simulink model "UAV_simple_hw_architecture"  (R2021b)
settings: Solver=VariableStepAuto  StartTime=0.0  StopTime=10.0  RelTol=1e-3
model workspace (MAT data in the model file):
  sensorData = Simulink.Bus
  sensorData.Alignment = -1
  sensorData.PreserveElementDimensions = 0
  sensorData.DataScope = 'Auto'
settings Model: Creator=esther  LastModifiedBy=esther

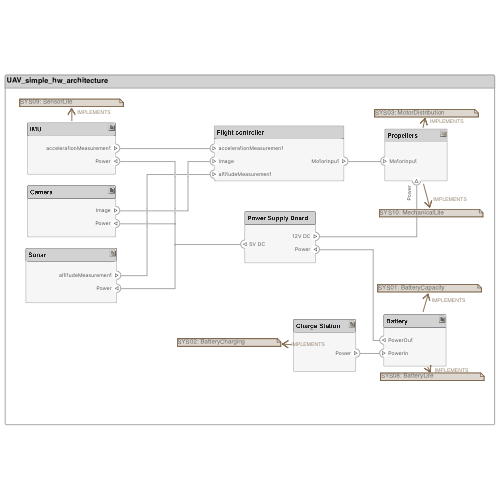
[thumbnail: Simulink's stored preview of the top-level diagram]
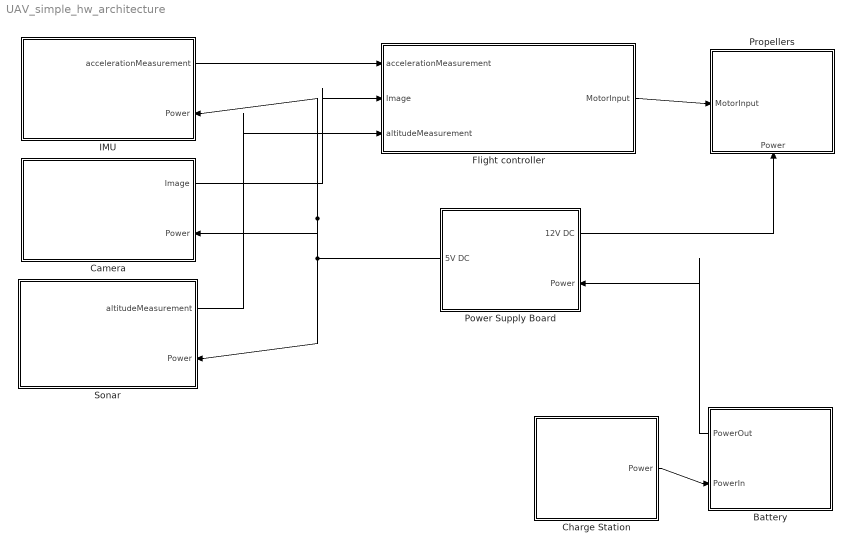
== system UAV_simple_hw_architecture ==
  Battery : Subsystem
      settings: PortSchema="{\"entries\":[{\"content\":{\"headerSize\":26,\"margin\":15,\"minimumSpacing\":25,\"sides\":[{\"content\":{\"connectorIds\":[\"Out1\",\"In1\"]},\"type\":\"ConnectorPlacement.EquallySpacedRectSide\",\"uuid\":\"982650e6-ddcc-430e-b118-190f1a8c1bc9\"},{\"content\":{\"connectorIds\":[],\"side\":\"RIGHT\"},\"type\":\"ConnectorPlacement.EquallySpacedRectSide\",\"uuid\":\"ed844e2c-e9bb-41b6-92bb-7e682fbb84b4\"},{\"content\":{\"connectorIds\":[],\"side\":\"TOP\"},\"type\":\"ConnectorPlacement.EquallySpacedRectSide\",\"uuid\":\"fdc513b0-7393-49dc-b7da-10bb51e0d5fd\"},{\"content\":{\"connectorIds\":[],\"side\":\"BOTTOM\"},\"type\":\"ConnectorPlacement.EquallySpacedRectSide\",\"uuid\":\"d8953aff-5649-44c5-a700-2c484cd66d11\"}]},\"type\":\"ConnectorPlacement.EquallySpacedConnector\",\"uuid\":\"3b6a0f0d-75bf-4e75-a7db-e0984288cb82\"}],\"packageUris\":[\"http://schema.mathworks.com/mf0/Connector/R2020b\"],\"version\":\"1.0\"}"
  Camera : Subsystem
      settings: PortSchema="{\"entries\":[{\"content\":{\"headerSize\":26,\"margin\":15,\"minimumSpacing\":25,\"sides\":[{\"content\":{\"connectorIds\":[]},\"type\":\"ConnectorPlacement.EquallySpacedRectSide\",\"uuid\":\"982650e6-ddcc-430e-b118-190f1a8c1bc9\"},{\"content\":{\"connectorIds\":[\"Out1\",\"In1\"],\"side\":\"RIGHT\"},\"type\":\"ConnectorPlacement.EquallySpacedRectSide\",\"uuid\":\"ed844e2c-e9bb-41b6-92bb-7e682fbb84b4\"},{\"content\":{\"connectorIds\":[],\"side\":\"TOP\"},\"type\":\"ConnectorPlacement.EquallySpacedRectSide\",\"uuid\":\"fdc513b0-7393-49dc-b7da-10bb51e0d5fd\"}]},\"type\":\"ConnectorPlacement.EquallySpacedConnector\",\"uuid\":\"3b6a0f0d-75bf-4e75-a7db-e0984288cb82\"}],\"packageUris\":[\"http://schema.mathworks.com/mf0/Connector/R2020b\"],\"version\":\"1.0\"}"
  Charge Station : Subsystem
      settings: PortSchema="{\"entries\":[{\"content\":{\"headerSize\":26,\"margin\":15,\"minimumSpacing\":25,\"sides\":[{\"content\":{\"connectorIds\":[]},\"type\":\"ConnectorPlacement.EquallySpacedRectSide\",\"uuid\":\"982650e6-ddcc-430e-b118-190f1a8c1bc9\"},{\"content\":{\"connectorIds\":[\"Out1\"],\"side\":\"RIGHT\"},\"type\":\"ConnectorPlacement.EquallySpacedRectSide\",\"uuid\":\"ed844e2c-e9bb-41b6-92bb-7e682fbb84b4\"},{\"content\":{\"connectorIds\":[],\"side\":\"TOP\"},\"type\":\"ConnectorPlacement.EquallySpacedRectSide\",\"uuid\":\"fdc513b0-7393-49dc-b7da-10bb51e0d5fd\"},{\"content\":{\"connectorIds\":[],\"side\":\"BOTTOM\"},\"type\":\"ConnectorPlacement.EquallySpacedRectSide\",\"uuid\":\"f65790e6-192e-4ff3-bd83-402d49a1232e\"}]},\"type\":\"ConnectorPlacement.EquallySpacedConnector\",\"uuid\":\"3b6a0f0d-75bf-4e75-a7db-e0984288cb82\"}],\"packageUris\":[\"http://schema.mathworks.com/mf0/Connector/R2020b\"],\"version\":\"1.0\"}"
  Flight controller : Subsystem
      settings: PortSchema="{\"entries\":[{\"content\":{\"headerSize\":26,\"margin\":15,\"minimumSpacing\":25,\"sides\":[{\"content\":{\"connectorIds\":[\"In1\",\"In2\",\"In3\"]},\"type\":\"ConnectorPlacement.EquallySpacedRectSide\",\"uuid\":\"982650e6-ddcc-430e-b118-190f1a8c1bc9\"},{\"content\":{\"connectorIds\":[\"Out1\"],\"side\":\"RIGHT\"},\"type\":\"ConnectorPlacement.EquallySpacedRectSide\",\"uuid\":\"ed844e2c-e9bb-41b6-92bb-7e682fbb84b4\"},{\"content\":{\"connectorIds\":[],\"side\":\"TOP\"},\"type\":\"ConnectorPlacement.EquallySpacedRectSide\",\"uuid\":\"fdc513b0-7393-49dc-b7da-10bb51e0d5fd\"}]},\"type\":\"ConnectorPlacement.EquallySpacedConnector\",\"uuid\":\"3b6a0f0d-75bf-4e75-a7db-e0984288cb82\"}],\"packageUris\":[\"http://schema.mathworks.com/mf0/Connector/R2020b\"],\"version\":\"1.0\"}"
  IMU : Subsystem
      settings: PortSchema="{\"entries\":[{\"content\":{\"headerSize\":26,\"margin\":15,\"minimumSpacing\":25,\"sides\":[{\"content\":{\"connectorIds\":[]},\"type\":\"ConnectorPlacement.EquallySpacedRectSide\",\"uuid\":\"982650e6-ddcc-430e-b118-190f1a8c1bc9\"},{\"content\":{\"connectorIds\":[\"Out1\",\"In1\"],\"side\":\"RIGHT\"},\"type\":\"ConnectorPlacement.EquallySpacedRectSide\",\"uuid\":\"ed844e2c-e9bb-41b6-92bb-7e682fbb84b4\"},{\"content\":{\"connectorIds\":[],\"side\":\"TOP\"},\"type\":\"ConnectorPlacement.EquallySpacedRectSide\",\"uuid\":\"fdc513b0-7393-49dc-b7da-10bb51e0d5fd\"}]},\"type\":\"ConnectorPlacement.EquallySpacedConnector\",\"uuid\":\"3b6a0f0d-75bf-4e75-a7db-e0984288cb82\"}],\"packageUris\":[\"http://schema.mathworks.com/mf0/Connector/R2020b\"],\"version\":\"1.0\"}"
  Power Supply Board : Subsystem
      settings: PortSchema="{\"entries\":[{\"content\":{\"headerSize\":26,\"margin\":15,\"minimumSpacing\":25,\"sides\":[{\"content\":{\"connectorIds\":[\"Out1\"]},\"type\":\"ConnectorPlacement.EquallySpacedRectSide\",\"uuid\":\"982650e6-ddcc-430e-b118-190f1a8c1bc9\"},{\"content\":{\"connectorIds\":[\"Out2\",\"In1\"],\"side\":\"RIGHT\"},\"type\":\"ConnectorPlacement.EquallySpacedRectSide\",\"uuid\":\"ed844e2c-e9bb-41b6-92bb-7e682fbb84b4\"},{\"content\":{\"connectorIds\":[],\"side\":\"TOP\"},\"type\":\"ConnectorPlacement.EquallySpacedRectSide\",\"uuid\":\"fdc513b0-7393-49dc-b7da-10bb51e0d5fd\"},{\"content\":{\"connectorIds\":[],\"side\":\"BOTTOM\"},\"type\":\"ConnectorPlacement.EquallySpacedRectSide\",\"uuid\":\"f8114367-592b-4080-bb32-3693e142188e\"}]},\"type\":\"ConnectorPlacement.EquallySpacedConnector\",\"uuid\":\"3b6a0f0d-75bf-4e75-a7db-e0984288cb82\"}],\"packageUris\":[\"http://schema.mathworks.com/mf0/Connector/R2020b\"],\"version\":\"1.0\"}"
  Propellers : Subsystem
      settings: PortSchema="{\"entries\":[{\"content\":{\"headerSize\":26,\"margin\":15,\"minimumSpacing\":25,\"sides\":[{\"content\":{\"connectorIds\":[\"In2\"]},\"type\":\"ConnectorPlacement.EquallySpacedRectSide\",\"uuid\":\"982650e6-ddcc-430e-b118-190f1a8c1bc9\"},{\"content\":{\"connectorIds\":[],\"side\":\"RIGHT\"},\"type\":\"ConnectorPlacement.EquallySpacedRectSide\",\"uuid\":\"ed844e2c-e9bb-41b6-92bb-7e682fbb84b4\"},{\"content\":{\"connectorIds\":[],\"side\":\"TOP\"},\"type\":\"ConnectorPlacement.EquallySpacedRectSide\",\"uuid\":\"fdc513b0-7393-49dc-b7da-10bb51e0d5fd\"},{\"content\":{\"connectorIds\":[\"In1\"],\"side\":\"BOTTOM\"},\"type\":\"ConnectorPlacement.EquallySpacedRectSide\",\"uuid\":\"52faec3f-ad3b-42ed-99b3-5c998984a52d\"}]},\"type\":\"ConnectorPlacement.EquallySpacedConnector\",\"uuid\":\"3b6a0f0d-75bf-4e75-a7db-e0984288cb82\"}],\"packageUris\":[\"http://schema.mathworks.com/mf0/Connector/R2020b\"],\"version\":\"1.0\"}"
  Sonar : Subsystem
      settings: PortSchema="{\"entries\":[{\"content\":{\"headerSize\":26,\"margin\":15,\"minimumSpacing\":25,\"sides\":[{\"content\":{\"connectorIds\":[]},\"type\":\"ConnectorPlacement.EquallySpacedRectSide\",\"uuid\":\"982650e6-ddcc-430e-b118-190f1a8c1bc9\"},{\"content\":{\"connectorIds\":[\"Out1\",\"In1\"],\"side\":\"RIGHT\"},\"type\":\"ConnectorPlacement.EquallySpacedRectSide\",\"uuid\":\"ed844e2c-e9bb-41b6-92bb-7e682fbb84b4\"},{\"content\":{\"connectorIds\":[],\"side\":\"TOP\"},\"type\":\"ConnectorPlacement.EquallySpacedRectSide\",\"uuid\":\"fdc513b0-7393-49dc-b7da-10bb51e0d5fd\"},{\"content\":{\"connectorIds\":[],\"side\":\"BOTTOM\"},\"type\":\"ConnectorPlacement.EquallySpacedRectSide\",\"uuid\":\"4d75345a-daea-4f99-8331-bf523ec34e8c\"}]},\"type\":\"ConnectorPlacement.EquallySpacedConnector\",\"uuid\":\"3b6a0f0d-75bf-4e75-a7db-e0984288cb82\"}],\"packageUris\":[\"http://schema.mathworks.com/mf0/Connector/R2020b\"],\"version\":\"1.0\"}"
  wires:
  Sonar/1(altitudeMeasurement) -> Flight controller/3(altitudeMeasurement)
  Camera/1(Image) -> Flight controller/2(Image)
  IMU/1(accelerationMeasurement) -> Flight controller/1(accelerationMeasurement)
  Flight controller/1(MotorInput) -> Propellers/2(MotorInput)
  Power Supply Board/2(12V DC) -> Propellers/1(Power)
  Power Supply Board/1(5V DC) -> Sonar/1(Power), IMU/1(Power), Camera/1(Power)
  Battery/1(PowerOut) -> Power Supply Board/1(Power)
  Charge Station/1(Power) -> Battery/1(PowerIn)

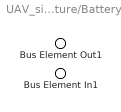
== system UAV_simple_hw_architecture/Battery ==
  Bus Element In1 : Inport  PortName=PowerIn
  Bus Element Out1 : Outport  PortName=PowerOut

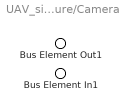
== system UAV_simple_hw_architecture/Camera ==
  Bus Element In1 : Inport  PortName=Power
  Bus Element Out1 : Outport  PortName=Image

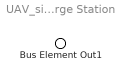
== system UAV_simple_hw_architecture/Charge Station ==
  Bus Element Out1 : Outport  PortName=Power

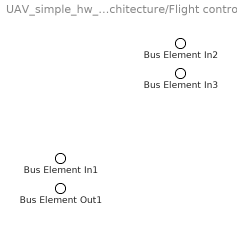
== system UAV_simple_hw_architecture/Flight controller ==
  Bus Element In3 : Inport  PortName=accelerationMeasurement
  Bus Element In2 : Inport  Port=2  PortName=Image
  Bus Element In1 : Inport  Port=3  PortName=altitudeMeasurement
  Bus Element Out1 : Outport  PortName=MotorInput

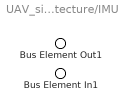
== system UAV_simple_hw_architecture/IMU ==
  Bus Element In1 : Inport  PortName=Power
  Bus Element Out1 : Outport  PortName=accelerationMeasurement

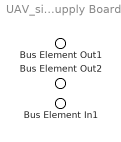
== system UAV_simple_hw_architecture/Power Supply Board ==
  Bus Element In1 : Inport  PortName=Power
  Bus Element Out1 : Outport  PortName=5V DC
  Bus Element Out2 : Outport  Port=2  PortName=12V DC

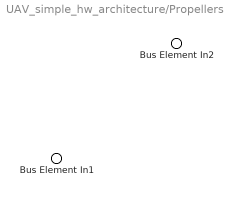
== system UAV_simple_hw_architecture/Propellers ==
  Bus Element In2 : Inport  PortName=Power
  Bus Element In1 : Inport  Port=2  PortName=MotorInput

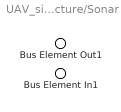
== system UAV_simple_hw_architecture/Sonar ==
  Bus Element In1 : Inport  PortName=Power
  Bus Element Out1 : Outport  PortName=altitudeMeasurement
